simulink model "bh_4bar_model_DYN"  (R2022b)
settings: Solver=ode45  StartTime=0.0  StopTime=10  FixedStep=0.001  MaxStep=0.1  RelTol=1e-9  AbsTol=1e-9  EnableMultiTasking=on
values from neighbouring files (symbols this model uses):
  L1 = 0.4    [bh_4bar_kin_z_analysis_CLS.m]
  L2 = 1.4    [bh_4bar_kin_z_analysis_CLS.m]
  L3 = 1.2    [bh_4bar_kin_z_analysis_CLS.m]
  L4 = 1    [bh_4bar_kin_z_analysis_CLS.m]
  N = length(THE_DEG_ANG_VEC)    [bh_4bar_kin_z_analysis_CLS.m]
  X = my_stuff_T.theta_deg_vec    [bh_4bar_kin_z_analysis_CLS.m]
undefined symbols (not defined in the file or in its folder): alpha_0_rad, alpha_dot_0_rad, alpha_rad, g, H, I_G1, I_G2, I_G3, m1, m2, m3, phi_0_rad, phi_dot_0_rad, phi_rad, theta_0_rad, theta_dot_0_rad, W, Y, Z
libraries: nesl_utility x20, sm_lib x15, simulink_extras x14, bh_4bar_SL_LIB x13
(part 2 of 3)

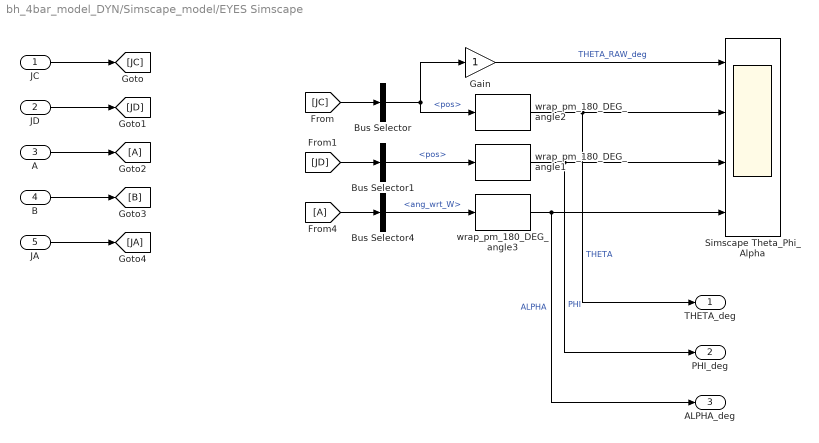
== system bh_4bar_model_DYN/Simscape_model/EYES Simscape ==
  JC : Inport
  JD : Inport  Port=2
  A : Inport  Port=3
  B : Inport  Port=4
  JA : Inport  Port=5
  Bus Selector : BusSelector  OutputSignals=pos
  Bus Selector1 : BusSelector  OutputSignals=pos
  Bus Selector4 : BusSelector  OutputSignals=ang_wrt_W
  From4 : From
  Gain : Gain
  Goto2 : Goto
  Simscape Theta_Phi_Alpha : Scope  NumInputPorts=4
  wrap_pm_180_DEG_angle1 : bh_4bar_SL_LIB/4bar_basics/wrap_pm_180_DEG_angle  SystemSampleTime=-1  VariantActivationTime=update diagram  Latency=0  AutoFrameSizeCalculation=off
  wrap_pm_180_DEG_angle2 : bh_4bar_SL_LIB/4bar_basics/wrap_pm_180_DEG_angle  SystemSampleTime=-1  VariantActivationTime=update diagram  Latency=0  AutoFrameSizeCalculation=off
  wrap_pm_180_DEG_angle3 : bh_4bar_SL_LIB/4bar_basics/wrap_pm_180_DEG_angle  SystemSampleTime=-1  VariantActivationTime=update diagram  Latency=0  AutoFrameSizeCalculation=off
  THETA_deg : Outport  VectorParamsAs1DForOutWhenUnconnected=off
  PHI_deg : Outport  Port=2  VectorParamsAs1DForOutWhenUnconnected=off
  ALPHA_deg : Outport  Port=3  VectorParamsAs1DForOutWhenUnconnected=off
  wires:
  B/1 -> [B]
  A/1 -> Goto2/1
  JD/1 -> [JD]
  JC/1 -> [JC]
  [JD] -> Bus Selector1/1
  [JC] -> Bus Selector/1
  Bus Selector/1 -> wrap_pm_180_DEG_angle2/1, Gain/1  "<pos>"
  From4/1 -> Bus Selector4/1
  wrap_pm_180_DEG_angle2/1 -> THETA_deg/1, Simscape Theta_Phi_Alpha/2  "THETA"
  wrap_pm_180_DEG_angle1/1 -> PHI_deg/1, Simscape Theta_Phi_Alpha/3  "PHI"
  JA/1 -> [JA]
  wrap_pm_180_DEG_angle3/1 -> ALPHA_deg/1, Simscape Theta_Phi_Alpha/4  "ALPHA"
  Gain/1 -> Simscape Theta_Phi_Alpha/1  "THETA_RAW_deg"
  Bus Selector1/1 -> wrap_pm_180_DEG_angle1/1  "<pos>"
  Bus Selector4/1 -> wrap_pm_180_DEG_angle3/1  "<ang_wrt_W>"

== system bh_4bar_model_DYN/Simscape_model/GROUND_C ==
  Mechanism Configuration : sm_lib/Utilities/Mechanism Configuration  UniformGravity=Constant  GravityVector="[0 -g  0]"  GravityUnits=m/s^2  LinearizationDelta=0.001  JointModeTransitionNonlinearIterations=2
  Solver Configuration : nesl_utility/Solver Configuration  PhysicalDomain=network_engine_domain  SubClassName=solver  LeftPortType=input  RightPortType=generic  Tones=[]  Harmonics=[]  SimulateNoise=off  Profile=off  UseLocalSampling=off  EnableSwitchedLinearOptims=on  FrequencyDomain=off  UseCCode=off  RelTol=0.001  AbsTol=1e-06  MinStep=1e-09  ToWorkspace=off  RevertToSquareIcSolve=off  NumHomotopyIterations=100  PhasorMode=off  PhasorModeNumHarmonics=1  ConsistencySolver=NEWTON_FTOL  IndexReductionMethod=DerivativeReplacement  DoDC=off  ResidualTolerance=1e-09  ConsistencyTolSource=GLOBAL  ConsistencyAbsTol=0.001  ConsistencyRelTol=0.001  ConsistencyTolFactor=0.001  UseLocalSolver=off  LocalSolverChoice=NE_BACKWARD_EULER_ADVANCER  ResolveIndetEquations=on  FunctionEvalNumThread=1  LocalSolverSampleTime=0.001  DoFixedCost=off  MaxNonlinIter=3  MaxModeIter=2  ComputeImpulses=off  ImpulseIterations=2  LinearAlgebra=Sparse  LinearAlgebraNumThread=0  EquationFormulation=NE_TIME_EF  DelaysMemoryBudget=1024  AutomaticFiltering=on  FilteringTimeConstant=0.001  PartitionStorageMethod=AS_NEEDED  PartitionMemoryBudget=1024  PartitionMethod=FAST
  World Frame : sm_lib/Frames and Transforms/World Frame
  Conn1 : PMIOPort  Side=Right
  connections:
  Solver Configuration/RConn1 -- Conn1/RConn1 -- Mechanism Configuration/RConn1 -- World Frame/RConn1

== system bh_4bar_model_DYN/Simscape_model/GROUND_D ==
  Rigid Transform : sm_lib/Frames and Transforms/Rigid Transform  TranslationMethod=StandardAxis  TranslationStandardOffset=L4  TranslationLengthUnit=m  TranslationStandardAxis=+X  TranslationCartesianOffset=[0 0 0]  TranslationROffset=0  TranslationROffsetUnits=m  TranslationZOffset=0  TranslationZOffsetUnits=m  TranslationThetaOffset=0  TranslationThetaOffsetUnits=deg  RotationMethod=None  RotationAngleUnits=deg  RotationStandardAxis=+Z  RotationAngle=0.0  RotationArbitraryAxis=[0 0 1]  FollAlignAxisA=+X  BaseAlignAxisA=+Y  FollAlignAxisB=+Y  BaseAlignAxisB=+Z  RotationSequenceAxes=FollowerAxes  RotationSequence=XYX  RotationSequenceAngles=[0 0 0]  RotationSequenceAnglesUnits=deg  RotationMatrix=[1 0 0; 0 1 0; 0 0 1]  Quaternion=[1 0 0 0]
  World Frame1 : sm_lib/Frames and Transforms/World Frame
  Conn1 : PMIOPort  Side=Right
  connections:
  Rigid Transform/LConn1 -- World Frame1/RConn1
  Rigid Transform/RConn1 -- Conn1/RConn1

== system bh_4bar_model_DYN/Simscape_model/Subsystem ==
  THETA_deg : Inport
  PHI_deg : Inport  Port=2
  ALPHA_deg : Inport  Port=3
  Bus Creator : BusCreator  Inputs=3
  ANG_BUS : Outport  VectorParamsAs1DForOutWhenUnconnected=off
  wires:
  ALPHA_deg/1 -> Bus Creator/3  "ALPHA_deg"
  PHI_deg/1 -> Bus Creator/2  "PHI_deg"
  THETA_deg/1 -> Bus Creator/1  "THETA_deg"
  Bus Creator/1 -> ANG_BUS/1

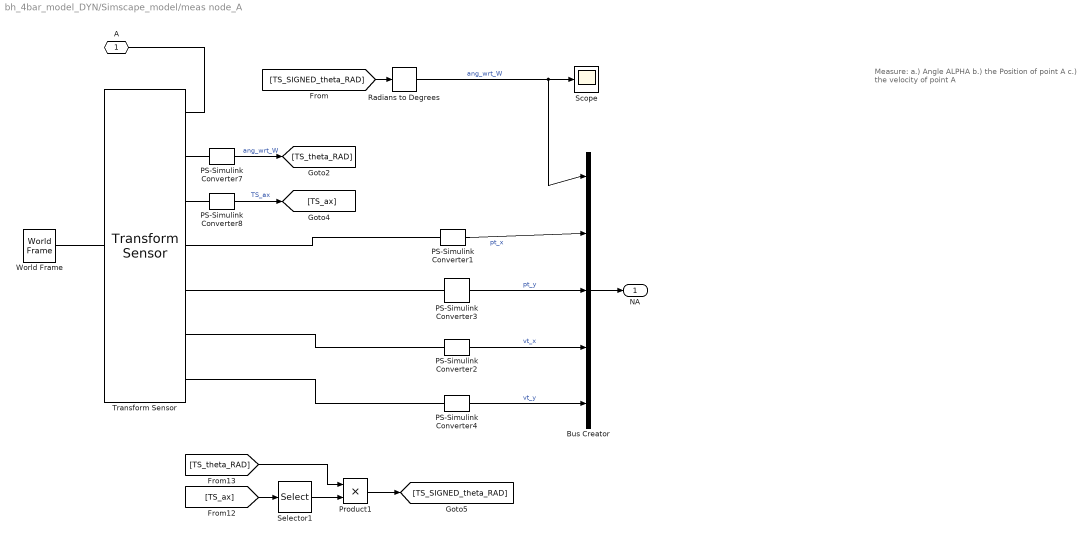
== system bh_4bar_model_DYN/Simscape_model/meas node_A ==
  note: Measure:
      | a.) Angle ALPHA
      | b.) the Position of point A
      | c.) the velocity of point A
  Bus Creator : BusCreator  Inputs=5
  PS-Simulink Converter1 : nesl_utility/PS-Simulink Converter  PhysicalDomain=network_engine_domain  SubClassName=ps_output  LeftPortType=input  RightPortType=output  PseudoPeriodic=off  Frequencies=[]  VectorFormat=1-D array  Unit=m  AffineConversion=off
      settings: AttributesFormatString=UNITS=%<Unit>
  PS-Simulink Converter2 : nesl_utility/PS-Simulink Converter  PhysicalDomain=network_engine_domain  SubClassName=ps_output  LeftPortType=input  RightPortType=output  PseudoPeriodic=off  Frequencies=[]  VectorFormat=1-D array  Unit=m/s  AffineConversion=off
      settings: AttributesFormatString=UNITS=%<Unit>
  PS-Simulink Converter3 : nesl_utility/PS-Simulink Converter  PhysicalDomain=network_engine_domain  SubClassName=ps_output  LeftPortType=input  RightPortType=output  PseudoPeriodic=off  Frequencies=[]  VectorFormat=1-D array  Unit=m  AffineConversion=off
      settings: AttributesFormatString=UNITS=%<Unit>
  PS-Simulink Converter4 : nesl_utility/PS-Simulink Converter  PhysicalDomain=network_engine_domain  SubClassName=ps_output  LeftPortType=input  RightPortType=output  PseudoPeriodic=off  Frequencies=[]  VectorFormat=1-D array  Unit=m/s  AffineConversion=off
      settings: AttributesFormatString=UNITS=%<Unit>
  PS-Simulink Converter7 : nesl_utility/PS-Simulink Converter  PhysicalDomain=network_engine_domain  SubClassName=ps_output  LeftPortType=input  RightPortType=output  PseudoPeriodic=off  Frequencies=[]  VectorFormat=1-D array  Unit=rad  AffineConversion=off
      settings: AttributesFormatString=UNITS=%<Unit>
  PS-Simulink Converter8 : nesl_utility/PS-Simulink Converter  PhysicalDomain=network_engine_domain  SubClassName=ps_output  LeftPortType=input  RightPortType=output  PseudoPeriodic=off  Frequencies=[]  VectorFormat=1-D array  Unit=1  AffineConversion=off
      settings: AttributesFormatString=UNITS=%<Unit>
  Product1 : Product
  Radians to Degrees : simulink_extras/Transformations/Radians to Degrees
  Scope : Scope
  Selector1 : Selector  InputPortWidth=3  IndexOptions=Index vector (dialog)  Indices=3  OutputSizes=1
  Transform Sensor : sm_lib/Frames and Transforms/Transform Sensor  MeasurementFrame=World  SenseAngle=on  SenseAxis=on  SenseQ=off  SenseR=off  SenseRotationSequence=off  RotationSequence=XYX  SenseOmegaX=off  SenseOmegaY=off  SenseOmegaZ=off  SenseQDot=off  SenseRDot=off  SenseAlphaX=off  SenseAlphaY=off  SenseAlphaZ=off  SenseQDDot=off  SenseRDDot=off  SenseX=on  SenseY=on  SenseZ=off  SenseRad=off  SenseAzim=off  SenseDist=off  SenseInc=off  SenseXDot=on  SenseYDot=on  SenseZDot=off  SenseRadDot=off  SenseAzimDot=off  SenseDistDot=off  SenseIncDot=off  SenseXDDot=off  SenseYDDot=off  SenseZDDot=off  SenseRadDDot=off  SenseAzimDDot=off  SenseDistDDot=off  SenseIncDDot=off
  World Frame : sm_lib/Frames and Transforms/World Frame
  A : PMIOPort  Side=Left
  NA : Outport  VectorParamsAs1DForOutWhenUnconnected=off
  wires:
  PS-Simulink Converter2/1 -> Bus Creator/4  "vt_x"
  Bus Creator/1 -> NA/1
  PS-Simulink Converter1/1 -> Bus Creator/2  "pt_x"
  PS-Simulink Converter4/1 -> Bus Creator/5  "vt_y"
  PS-Simulink Converter3/1 -> Bus Creator/3  "pt_y"
  Radians to Degrees/1 -> Bus Creator/1, Scope/1  "ang_wrt_W"
  [TS_theta_RAD] -> Product1/1
  [TS_ax] -> Selector1/1
  Product1/1 -> [TS_SIGNED_theta_RAD]
  Selector1/1 -> Product1/2
  PS-Simulink Converter7/1 -> [TS_theta_RAD]  "ang_wrt_W"
  PS-Simulink Converter8/1 -> [TS_ax]  "TS_ax"
  [TS_SIGNED_theta_RAD] -> Radians to Degrees/1
  connections:
  A/RConn1 -- Transform Sensor/RConn1
  Transform Sensor/LConn1 -- World Frame/RConn1
  Transform Sensor/RConn7 -- PS-Simulink Converter4/LConn1
  PS-Simulink Converter2/LConn1 -- Transform Sensor/RConn6
  PS-Simulink Converter3/LConn1 -- Transform Sensor/RConn5
  PS-Simulink Converter1/LConn1 -- Transform Sensor/RConn4
  PS-Simulink Converter7/LConn1 -- Transform Sensor/RConn2
  PS-Simulink Converter8/LConn1 -- Transform Sensor/RConn3

== system bh_4bar_model_DYN/Simscape_model/meas node_A1 ==
  note: Measure:
      | a.) Angle ALPHA
      | b.) the Position of point A
      | c.) the velocity of point A
  Bus Creator : BusCreator  Inputs=5
  PS-Simulink Converter1 : nesl_utility/PS-Simulink Converter  PhysicalDomain=network_engine_domain  SubClassName=ps_output  LeftPortType=input  RightPortType=output  PseudoPeriodic=off  Frequencies=[]  VectorFormat=1-D array  Unit=m  AffineConversion=off
      settings: AttributesFormatString=UNITS=%<Unit>
  PS-Simulink Converter2 : nesl_utility/PS-Simulink Converter  PhysicalDomain=network_engine_domain  SubClassName=ps_output  LeftPortType=input  RightPortType=output  PseudoPeriodic=off  Frequencies=[]  VectorFormat=1-D array  Unit=m/s  AffineConversion=off
      settings: AttributesFormatString=UNITS=%<Unit>
  PS-Simulink Converter3 : nesl_utility/PS-Simulink Converter  PhysicalDomain=network_engine_domain  SubClassName=ps_output  LeftPortType=input  RightPortType=output  PseudoPeriodic=off  Frequencies=[]  VectorFormat=1-D array  Unit=m  AffineConversion=off
      settings: AttributesFormatString=UNITS=%<Unit>
  PS-Simulink Converter4 : nesl_utility/PS-Simulink Converter  PhysicalDomain=network_engine_domain  SubClassName=ps_output  LeftPortType=input  RightPortType=output  PseudoPeriodic=off  Frequencies=[]  VectorFormat=1-D array  Unit=m/s  AffineConversion=off
      settings: AttributesFormatString=UNITS=%<Unit>
  PS-Simulink Converter7 : nesl_utility/PS-Simulink Converter  PhysicalDomain=network_engine_domain  SubClassName=ps_output  LeftPortType=input  RightPortType=output  PseudoPeriodic=off  Frequencies=[]  VectorFormat=1-D array  Unit=rad  AffineConversion=off
      settings: AttributesFormatString=UNITS=%<Unit>
  PS-Simulink Converter8 : nesl_utility/PS-Simulink Converter  PhysicalDomain=network_engine_domain  SubClassName=ps_output  LeftPortType=input  RightPortType=output  PseudoPeriodic=off  Frequencies=[]  VectorFormat=1-D array  Unit=1  AffineConversion=off
      settings: AttributesFormatString=UNITS=%<Unit>
  Product1 : Product
  Radians to Degrees : simulink_extras/Transformations/Radians to Degrees
  Scope : Scope
  Selector1 : Selector  InputPortWidth=3  IndexOptions=Index vector (dialog)  Indices=3  OutputSizes=1
  Transform Sensor : sm_lib/Frames and Transforms/Transform Sensor  MeasurementFrame=World  SenseAngle=on  SenseAxis=on  SenseQ=off  SenseR=off  SenseRotationSequence=off  RotationSequence=XYX  SenseOmegaX=off  SenseOmegaY=off  SenseOmegaZ=off  SenseQDot=off  SenseRDot=off  SenseAlphaX=off  SenseAlphaY=off  SenseAlphaZ=off  SenseQDDot=off  SenseRDDot=off  SenseX=on  SenseY=on  SenseZ=off  SenseRad=off  SenseAzim=off  SenseDist=off  SenseInc=off  SenseXDot=on  SenseYDot=on  SenseZDot=off  SenseRadDot=off  SenseAzimDot=off  SenseDistDot=off  SenseIncDot=off  SenseXDDot=off  SenseYDDot=off  SenseZDDot=off  SenseRadDDot=off  SenseAzimDDot=off  SenseDistDDot=off  SenseIncDDot=off
  World Frame : sm_lib/Frames and Transforms/World Frame
  B : PMIOPort  Side=Left
  NB : Outport  VectorParamsAs1DForOutWhenUnconnected=off
  wires:
  PS-Simulink Converter2/1 -> Bus Creator/4  "vt_x"
  Bus Creator/1 -> NB/1
  PS-Simulink Converter1/1 -> Bus Creator/2  "pt_x"
  PS-Simulink Converter4/1 -> Bus Creator/5  "vt_y"
  PS-Simulink Converter3/1 -> Bus Creator/3  "pt_y"
  Radians to Degrees/1 -> Bus Creator/1, Scope/1  "ang_wrt_W"
  [TS_theta_RAD] -> Product1/1
  [TS_ax] -> Selector1/1
  Product1/1 -> [TS_SIGNED_theta_RAD]
  Selector1/1 -> Product1/2
  PS-Simulink Converter7/1 -> [TS_theta_RAD]  "ang_wrt_W"
  PS-Simulink Converter8/1 -> [TS_ax]  "TS_ax"
  [TS_SIGNED_theta_RAD] -> Radians to Degrees/1
  connections:
  B/RConn1 -- Transform Sensor/RConn1
  Transform Sensor/LConn1 -- World Frame/RConn1
  Transform Sensor/RConn7 -- PS-Simulink Converter4/LConn1
  PS-Simulink Converter2/LConn1 -- Transform Sensor/RConn6
  PS-Simulink Converter3/LConn1 -- Transform Sensor/RConn5
  PS-Simulink Converter1/LConn1 -- Transform Sensor/RConn4
  PS-Simulink Converter7/LConn1 -- Transform Sensor/RConn2
  PS-Simulink Converter8/LConn1 -- Transform Sensor/RConn3

== system bh_4bar_model_DYN/Simscape_model/meas_JA ==
  Bus Creator : BusCreator  Inputs=2
  PS-Simulink Converter1 : nesl_utility/PS-Simulink Converter  PhysicalDomain=network_engine_domain  SubClassName=ps_output  LeftPortType=input  RightPortType=output  PseudoPeriodic=off  Frequencies=[]  VectorFormat=1-D array  Unit=deg  AffineConversion=off
  PS-Simulink Converter2 : nesl_utility/PS-Simulink Converter  PhysicalDomain=network_engine_domain  SubClassName=ps_output  LeftPortType=input  RightPortType=output  PseudoPeriodic=off  Frequencies=[]  VectorFormat=1-D array  Unit=deg/s  AffineConversion=off
  q : PMIOPort  Side=Left
  w : PMIOPort  Port=2  Side=Left
  PV_BUS : Outport  VectorParamsAs1DForOutWhenUnconnected=off
  wires:
  PS-Simulink Converter2/1 -> Bus Creator/2  "vel"
  PS-Simulink Converter1/1 -> Bus Creator/1  "pos"
  Bus Creator/1 -> PV_BUS/1
  connections:
  q/RConn1 -- PS-Simulink Converter1/LConn1
  PS-Simulink Converter2/LConn1 -- w/RConn1

== system bh_4bar_model_DYN/Simscape_model/meas_JC ==
  Bus Creator : BusCreator  Inputs=2
  PS-Simulink Converter1 : nesl_utility/PS-Simulink Converter  PhysicalDomain=network_engine_domain  SubClassName=ps_output  LeftPortType=input  RightPortType=output  PseudoPeriodic=off  Frequencies=[]  VectorFormat=1-D array  Unit=deg  AffineConversion=off
      settings: AttributesFormatString=UNITS=%<Unit>
  PS-Simulink Converter2 : nesl_utility/PS-Simulink Converter  PhysicalDomain=network_engine_domain  SubClassName=ps_output  LeftPortType=input  RightPortType=output  PseudoPeriodic=off  Frequencies=[]  VectorFormat=1-D array  Unit=deg/s  AffineConversion=off
      settings: AttributesFormatString=UNITS=%<Unit>
  q : PMIOPort  Side=Left
  w : PMIOPort  Port=2  Side=Left
  PV_BUS : Outport  VectorParamsAs1DForOutWhenUnconnected=off
  wires:
  PS-Simulink Converter2/1 -> Bus Creator/2  "vel"
  PS-Simulink Converter1/1 -> Bus Creator/1  "pos"
  Bus Creator/1 -> PV_BUS/1
  connections:
  q/RConn1 -- PS-Simulink Converter1/LConn1
  PS-Simulink Converter2/LConn1 -- w/RConn1

== system bh_4bar_model_DYN/Simscape_model/meas_JD ==
  Bus Creator : BusCreator  Inputs=2
  PS-Simulink Converter1 : nesl_utility/PS-Simulink Converter  PhysicalDomain=network_engine_domain  SubClassName=ps_output  LeftPortType=input  RightPortType=output  PseudoPeriodic=off  Frequencies=[]  VectorFormat=1-D array  Unit=deg  AffineConversion=off
  PS-Simulink Converter2 : nesl_utility/PS-Simulink Converter  PhysicalDomain=network_engine_domain  SubClassName=ps_output  LeftPortType=input  RightPortType=output  PseudoPeriodic=off  Frequencies=[]  VectorFormat=1-D array  Unit=deg/s  AffineConversion=off
  q : PMIOPort  Side=Left
  w : PMIOPort  Port=2  Side=Left
  PV_BUS : Outport  VectorParamsAs1DForOutWhenUnconnected=off
  wires:
  PS-Simulink Converter2/1 -> Bus Creator/2  "vel"
  PS-Simulink Converter1/1 -> Bus Creator/1  "pos"
  Bus Creator/1 -> PV_BUS/1
  connections:
  q/RConn1 -- PS-Simulink Converter1/LConn1
  PS-Simulink Converter2/LConn1 -- w/RConn1

== matlab function bh_4bar_model_DYN/Hand_model/THE_THETA_SYS_DD ==
  data: I_G1 input; theta_DD output; I_G2 input; I_G3 input; L_1 input; L_2 input; L_3 input; alpha input; g input; m_1 input; m_2 input; m_3 input; phi input; tau_1 input; theta input; theta_dot input
function theta_DD = THE_THETA_SYS_DD(I_G1,I_G2,I_G3,L_1,L_2,L_3,alpha,g,m_1,m_2,m_3,phi,tau_1,theta,theta_dot)
%#codegen

%    This function was generated by the Symbolic Math Toolbox version 9.2.
%    27-Oct-2022 15:33:01

et1 = I_G1+I_G3.*((L_1.*cos(alpha).*sin(theta))./(L_3.*(cos(alpha).*sin(phi)-cos(phi).*sin(alpha)))-(L_1.*sin(alpha).*cos(theta))./(L_3.*(cos(alpha).*sin(phi)-cos(phi).*sin(alpha)))).^2+I_G2.*((L_1.*cos(phi).*sin(theta))./(L_2.*(cos(alpha).*sin(phi)-cos(phi).*sin(alpha)))-(L_1.*cos(theta).*sin(phi))./(L_2.*(cos(alpha).*sin(phi)-cos(phi).*sin(alpha)))).^2;
et2 = (m_2.*((L_2.^2.*((L_1.*cos(phi).*sin(theta))./(L_2.*(cos(alpha).*sin(phi)-cos(phi).*sin(alpha)))-(L_1.*cos(theta).*sin(phi))./(L_2.*(cos(alpha).*sin(phi)-cos(phi).*sin(alpha)))).^2)./2.0+L_1.^2.*2.0+L_1.*L_2.*((L_1.*cos(phi).*sin(theta))./(L_2.*(cos(alpha).*sin(phi)-cos(phi).*sin(alpha)))-(L_1.*cos(theta).*sin(phi))./(L_2.*(cos(alpha).*sin(phi)-cos(phi).*sin(alpha)))).*(sin(alpha).*sin(theta)+cos(alpha).*cos(theta)).*2.0))./2.0+(L_1.^2.*m_1)./4.0;
et3 = (L_3.^2.*m_3.*((L_1.*cos(alpha).*sin(theta))./(L_3.*(cos(alpha).*sin(phi)-cos(phi).*sin(alpha)))-(L_1.*sin(alpha).*cos(theta))./(L_3.*(cos(alpha).*sin(phi)-cos(phi).*sin(alpha)))).^2)./4.0;
et4 = cos(alpha).*cos(phi).*((L_1.*cos(phi).*sin(theta))./(L_2.*(cos(alpha).*sin(phi)-cos(phi).*sin(alpha)))-(L_1.*cos(theta).*sin(phi))./(L_2.*(cos(alpha).*sin(phi)-cos(phi).*sin(alpha))))-sin(alpha).*sin(phi).*((L_1.*cos(alpha).*sin(theta))./(L_3.*(cos(alpha).*sin(phi)-cos(phi).*sin(alpha)))-(L_1.*sin(alpha).*cos(theta))./(L_3.*(cos(alpha).*sin(phi)-cos(phi).*sin(alpha))))+sin(alpha).*sin(phi).*((L_1.*cos(phi).*sin(theta))./(L_2.*(cos(alpha).*sin(phi)-cos(phi).*sin(alpha)))-(L_1.*cos(theta).*sin(phi))./(L_2.*(cos(alpha).*sin(phi)-cos(phi).*sin(alpha))));
et5 = -cos(alpha).*cos(phi).*((L_1.*cos(alpha).*sin(theta))./(L_3.*(cos(alpha).*sin(phi)-cos(phi).*sin(alpha)))-(L_1.*sin(alpha).*cos(theta))./(L_3.*(cos(alpha).*sin(phi)-cos(phi).*sin(alpha))));
et6 = cos(alpha).*cos(phi).*((L_1.*cos(phi).*sin(theta))./(L_2.*(cos(alpha).*sin(phi)-cos(phi).*sin(alpha)))-(L_1.*cos(theta).*sin(phi))./(L_2.*(cos(alpha).*sin(phi)-cos(phi).*sin(alpha))))-sin(alpha).*sin(phi).*((L_1.*cos(alpha).*sin(theta))./(L_3.*(cos(alpha).*sin(phi)-cos(phi).*sin(alpha)))-(L_1.*sin(alpha).*cos(theta))./(L_3.*(cos(alpha).*sin(phi)-cos(phi).*sin(alpha))))+sin(alpha).*sin(phi).*((L_1.*cos(phi).*sin(theta))./(L_2.*(cos(alpha).*sin(phi)-cos(phi).*sin(alpha)))-(L_1.*cos(theta).*sin(phi))./(L_2.*(cos(alpha).*sin(phi)-cos(phi).*sin(alpha))));
et7 = -cos(alpha).*cos(phi).*((L_1.*cos(alpha).*sin(theta))./(L_3.*(cos(alpha).*sin(phi)-cos(phi).*sin(alpha)))-(L_1.*sin(alpha).*cos(theta))./(L_3.*(cos(alpha).*sin(phi)-cos(phi).*sin(alpha))));
et8 = (L_1.*cos(phi).*cos(theta))./(L_2.*(cos(alpha).*sin(phi)-cos(phi).*sin(alpha)))+(L_1.*sin(phi).*sin(theta))./(L_2.*(cos(alpha).*sin(phi)-cos(phi).*sin(alpha)))+(L_1.*cos(phi).*sin(theta).*1.0./(cos(alpha).*sin(phi)-cos(phi).*sin(alpha)).^2.*(et4+et5))./L_2-(L_1.*cos(theta).*sin(phi).*1.0./(cos(alpha).*sin(phi)-cos(phi).*sin(alpha)).^2.*(et6+et7))./L_2-(L_1.*cos(phi).*cos(theta).*((L_1.*cos(alpha).*sin(theta))./(L_3.*(cos(alpha).*sin(phi)-cos(phi).*sin(alpha)))-(L_1.*sin(alpha).*cos(theta))./(L_3.*(cos(alpha).*sin(phi)-cos(phi).*sin(alpha)))))./(L_2.*(cos(alpha).*sin(phi)-cos(phi).*sin(alpha)));
et9 = -(L_1.*sin(phi).*sin(theta).*((L_1.*cos(alpha).*sin(theta))./(L_3.*(cos(alpha).*sin(phi)-cos(phi).*sin(alpha)))-(L_1.*sin(alpha).*cos(theta))./(L_3.*(cos(alpha).*sin(phi)-cos(phi).*sin(alpha)))))./(L_2.*(cos(alpha).*sin(phi)-cos(phi).*sin(alpha)));
et10 = cos(alpha).*cos(phi).*((L_1.*cos(phi).*sin(theta))./(L_2.*(cos(alpha).*sin(phi)-cos(phi).*sin(alpha)))-(L_1.*cos(theta).*sin(phi))./(L_2.*(cos(alpha).*sin(phi)-cos(phi).*sin(alpha))))-sin(alpha).*sin(phi).*((L_1.*cos(alpha).*sin(theta))./(L_3.*(cos(alpha).*sin(phi)-cos(phi).*sin(alpha)))-(L_1.*sin(alpha).*cos(theta))./(L_3.*(cos(alpha).*sin(phi)-cos(phi).*sin(alpha))))+sin(alpha).*sin(phi).*((L_1.*cos(phi).*sin(theta))./(L_2.*(cos(alpha).*sin(phi)-cos(phi).*sin(alpha)))-(L_1.*cos(theta).*sin(phi))./(L_2.*(cos(alpha).*sin(phi)-cos(phi).*sin(alpha))));
et11 = -cos(alpha).*cos(phi).*((L_1.*cos(alpha).*sin(theta))./(L_3.*(cos(alpha).*sin(phi)-cos(phi).*sin(alpha)))-(L_1.*sin(alpha).*cos(theta))./(L_3.*(cos(alpha).*sin(phi)-cos(phi).*sin(alpha))));
et12 = cos(alpha).*cos(phi).*((L_1.*cos(phi).*sin(theta))./(L_2.*(cos(alpha).*sin(phi)-cos(phi).*sin(alpha)))-(L_1.*cos(theta).*sin(phi))./(L_2.*(cos(alpha).*sin(phi)-cos(phi).*sin(alpha))))-sin(alpha).*sin(phi).*((L_1.*cos(alpha).*sin(theta))./(L_3.*(cos(alpha).*sin(phi)-cos(phi).*sin(alpha)))-(L_1.*sin(alpha).*cos(theta))./(L_3.*(cos(alpha).*sin(phi)-cos(phi).*sin(alpha))))+sin(alpha).*sin(phi).*((L_1.*cos(phi).*sin(theta))./(L_2.*(cos(alpha).*sin(phi)-cos(phi).*sin(alpha)))-(L_1.*cos(theta).*sin(phi))./(L_2.*(cos(alpha).*sin(phi)-cos(phi).*sin(alpha))));
et13 = -cos(alpha).*cos(phi).*((L_1.*cos(alpha).*sin(theta))./(L_3.*(cos(alpha).*sin(phi)-cos(phi).*sin(alpha)))-(L_1.*sin(alpha).*cos(theta))./(L_3.*(cos(alpha).*sin(phi)-cos(phi).*sin(alpha))));
et14 = (L_1.*cos(phi).*cos(theta))./(L_2.*(cos(alpha).*sin(phi)-cos(phi).*sin(alpha)))+(L_1.*sin(phi).*sin(theta))./(L_2.*(cos(alpha).*sin(phi)-cos(phi).*sin(alpha)))+(L_1.*cos(phi).*sin(theta).*1.0./(cos(alpha).*sin(phi)-cos(phi).*sin(alpha)).^2.*(et10+et11))./L_2-(L_1.*cos(theta).*sin(phi).*1.0./(cos(alpha).*sin(phi)-cos(phi).*sin(alpha)).^2.*(et12+et13))./L_2-(L_1.*cos(phi).*cos(theta).*((L_1.*cos(alpha).*sin(theta))./(L_3.*(cos(alpha).*sin(phi)-cos(phi).*sin(alpha)))-(L_1.*sin(alpha).*cos(theta))./(L_3.*(cos(alpha).*sin(phi)-cos(phi).*sin(alpha)))))./(L_2.*(cos(alpha).*sin(phi)-cos(phi).*sin(alpha)));
et15 = -(L_1.*sin(phi).*sin(theta).*((L_1.*cos(alpha).*sin(theta))./(L_3.*(cos(alpha).*sin(phi)-cos(phi).*sin(alpha)))-(L_1.*sin(alpha).*cos(theta))./(L_3.*(cos(alpha).*sin(phi)-cos(phi).*sin(alpha)))))./(L_2.*(cos(alpha).*sin(phi)-cos(phi).*sin(alpha)));
et16 = (L_2.^2.*theta_dot.^2.*((L_1.*cos(phi).*sin(theta))./(L_2.*(cos(alpha).*sin(phi)-cos(phi).*sin(alpha)))-(L_1.*cos(theta).*sin(phi))./(L_2.*(cos(alpha).*sin(phi)-cos(phi).*sin(alpha)))).*(et8+et9))./2.0+L_1.*L_2.*theta_dot.^2.*(sin(alpha).*sin(theta)+cos(alpha).*cos(theta)).*(et14+et15);
et17 = -L_1.*L_2.*theta_dot.^2.*((L_1.*cos(phi).*sin(theta))./(L_2.*(cos(alpha).*sin(phi)-cos(phi).*sin(alpha)))-(L_1.*cos(theta).*sin(phi))./(L_2.*(cos(alpha).*sin(phi)-cos(phi).*sin(alpha)))).*(cos(alpha).*sin(theta)-sin(alpha).*cos(theta)-cos(alpha).*sin(theta).*((L_1.*cos(phi).*sin(theta))./(L_2.*(cos(alpha).*sin(phi)-cos(phi).*sin(alpha)))-(L_1.*cos(theta).*sin(phi))./(L_2.*(cos(alpha).*sin(phi)-cos(phi).*sin(alpha))))+sin(alpha).*cos(theta).*((L_1.*cos(phi).*sin(theta))./(L_2.*(cos(alpha).*sin(phi)-cos(phi).*sin(alpha)))-(L_1.*cos(theta).*sin(phi))./(L_2.*(cos(alpha).*sin(phi)-cos(phi).*sin(alpha)))));
et18 = theta_dot.*cos(alpha).*cos(phi).*((L_1.*cos(alpha).*sin(theta))./(L_3.*(cos(alpha).*sin(phi)-cos(phi).*sin(alpha)))-(L_1.*sin(alpha).*cos(theta))./(L_3.*(cos(alpha).*sin(phi)-cos(phi).*sin(alpha))))-theta_dot.*cos(alpha).*cos(phi).*((L_1.*cos(phi).*sin(theta))./(L_2.*(cos(alpha).*sin(phi)-cos(phi).*sin(alpha)))-(L_1.*cos(theta).*sin(phi))./(L_2.*(cos(alpha).*sin(phi)-cos(phi).*sin(alpha))))+theta_dot.*sin(alpha).*sin(phi).*((L_1.*cos(alpha).*sin(theta))./(L_3.*(cos(alpha).*sin(phi)-cos(phi).*sin(alpha)))-(L_1.*sin(alpha).*cos(theta))./(L_3.*(cos(alpha).*sin(phi)-cos(phi).*sin(alpha))));
et19 = -theta_dot.*sin(alpha).*sin(phi).*((L_1.*cos(phi).*sin(theta))./(L_2.*(cos(alpha).*sin(phi)-cos(phi).*sin(alpha)))-(L_1.*cos(theta).*sin(phi))./(L_2.*(cos(alpha).*sin(phi)-cos(phi).*sin(alpha))));
et20 = theta_dot.*cos(alpha).*cos(phi).*((L_1.*cos(alpha).*sin(theta))./(L_3.*(cos(alpha).*sin(phi)-cos(phi).*sin(alpha)))-(L_1.*sin(alpha).*cos(theta))./(L_3.*(cos(alpha).*sin(phi)-cos(phi).*sin(alpha))))-theta_dot.*cos(alpha).*cos(phi).*((L_1.*cos(phi).*sin(theta))./(L_2.*(cos(alpha).*sin(phi)-cos(phi).*sin(alpha)))-(L_1.*cos(theta).*sin(phi))./(L_2.*(cos(alpha).*sin(phi)-cos(phi).*sin(alpha))))+theta_dot.*sin(alpha).*sin(phi).*((L_1.*cos(alpha).*sin(theta))./(L_3.*(cos(alpha).*sin(phi)-cos(phi).*sin(alpha)))-(L_1.*sin(alpha).*cos(theta))./(L_3.*(cos(alpha).*sin(phi)-cos(phi).*sin(alpha))));
et21 = -theta_dot.*sin(alpha).*sin(phi).*((L_1.*cos(phi).*sin(theta))./(L_2.*(cos(alpha).*sin(phi)-cos(phi).*sin(alpha)))-(L_1.*cos(theta).*sin(phi))./(L_2.*(cos(alpha).*sin(phi)-cos(phi).*sin(alpha))));
et22 = (L_1.*theta_dot.*cos(phi).*cos(theta))./(L_2.*(cos(alpha).*sin(phi)-cos(phi).*sin(alpha)))+(L_1.*theta_dot.*sin(phi).*sin(theta))./(L_2.*(cos(alpha).*sin(phi)-cos(phi).*sin(alpha)))-(L_1.*cos(phi).*sin(theta).*1.0./(cos(alpha).*sin(phi)-cos(phi).*sin(alpha)).^2.*(et18+et19))./L_2+(L_1.*cos(theta).*sin(phi).*1.0./(cos(alpha).*sin(phi)-cos(phi).*sin(alpha)).^2.*(et20+et21))./L_2-(L_1.*theta_dot.*cos(phi).*cos(theta).*((L_1.*cos(alpha).*sin(theta))./(L_3.*(cos(alpha).*sin(phi)-cos(phi).*sin(alpha)))-(L_1.*sin(alpha).*cos(theta))./(L_3.*(cos(alpha).*sin(phi)-cos(phi).*sin(alpha)))))./(L_2.*(cos(alpha).*sin(phi)-cos(phi).*sin(alpha)));
et23 = -(L_1.*theta_dot.*sin(phi).*sin(theta).*((L_1.*cos(alpha).*sin(theta))./(L_3.*(cos(alpha).*sin(phi)-cos(phi).*sin(alpha)))-(L_1.*sin(alpha).*cos(theta))./(L_3.*(cos(alpha).*sin(phi)-cos(phi).*sin(alpha)))))./(L_2.*(cos(alpha).*sin(phi)-cos(phi).*sin(alpha)));
et24 = theta_dot.*cos(alpha).*cos(phi).*((L_1.*cos(alpha).*sin(theta))./(L_3.*(cos(alpha).*sin(phi)-cos(phi).*sin(alpha)))-(L_1.*sin(alpha).*cos(theta))./(L_3.*(cos(alpha).*sin(phi)-cos(phi).*sin(alpha))))-theta_dot.*cos(alpha).*cos(phi).*((L_1.*cos(phi).*sin(theta))./(L_2.*(cos(alpha).*sin(phi)-cos(phi).*sin(alpha)))-(L_1.*cos(theta).*sin(phi))./(L_2.*(cos(alpha).*sin(phi)-cos(phi).*sin(alpha))))+theta_dot.*sin(alpha).*sin(phi).*((L_1.*cos(alpha).*sin(theta))./(L_3.*(cos(alpha).*sin(phi)-cos(phi).*sin(alpha)))-(L_1.*sin(alpha).*cos(theta))./(L_3.*(cos(alpha).*sin(phi)-cos(phi).*sin(alpha))));
et25 = -theta_dot.*sin(alpha).*sin(phi).*((L_1.*cos(phi).*sin(theta))./(L_2.*(cos(alpha).*sin(phi)-cos(phi).*sin(alpha)))-(L_1.*cos(theta).*sin(phi))./(L_2.*(cos(alpha).*sin(phi)-cos(phi).*sin(alpha))));
et26 = theta_dot.*cos(alpha).*cos(phi).*((L_1.*cos(alpha).*sin(theta))./(L_3.*(cos(alpha).*sin(phi)-cos(phi).*sin(alpha)))-(L_1.*sin(alpha).*cos(theta))./(L_3.*(cos(alpha).*sin(phi)-cos(phi).*sin(alpha))))-theta_dot.*cos(alpha).*cos(phi).*((L_1.*cos(phi).*sin(theta))./(L_2.*(cos(alpha).*sin(phi)-cos(phi).*sin(alpha)))-(L_1.*cos(theta).*sin(phi))./(L_2.*(cos(alpha).*sin(phi)-cos(phi).*sin(alpha))))+theta_dot.*sin(alpha).*sin(phi).*((L_1.*cos(alpha).*sin(theta))./(L_3.*(cos(alpha).*sin(phi)-cos(phi).*sin(alpha)))-(L_1.*sin(alpha).*cos(theta))./(L_3.*(cos(alpha).*sin(phi)-cos(phi).*sin(alpha))));
et27 = -theta_dot.*sin(alpha).*sin(phi).*((L_1.*cos(phi).*sin(theta))./(L_2.*(cos(alpha).*sin(phi)-cos(phi).*sin(alpha)))-(L_1.*cos(theta).*sin(phi))./(L_2.*(cos(alpha).*sin(phi)-cos(phi).*sin(alpha))));
et28 = (L_1.*theta_dot.*cos(phi).*cos(theta))./(L_2.*(cos(alpha).*sin(phi)-cos(phi).*sin(alpha)))+(L_1.*theta_dot.*sin(phi).*sin(theta))./(L_2.*(cos(alpha).*sin(phi)-cos(phi).*sin(alpha)))-(L_1.*cos(phi).*sin(theta).*1.0./(cos(alpha).*sin(phi)-cos(phi).*sin(alpha)).^2.*(et24+et25))./L_2+(L_1.*cos(theta).*sin(phi).*1.0./(cos(alpha).*sin(phi)-cos(phi).*sin(alpha)).^2.*(et26+et27))./L_2-(L_1.*theta_dot.*cos(phi).*cos(theta).*((L_1.*cos(alpha).*sin(theta))./(L_3.*(cos(alpha).*sin(phi)-cos(phi).*sin(alpha)))-(L_1.*sin(alpha).*cos(theta))./(L_3.*(cos(alpha).*sin(phi)-cos(phi).*sin(alpha)))))./(L_2.*(cos(alpha).*sin(phi)-cos(phi).*sin(alpha)));
et29 = -(L_1.*theta_dot.*sin(phi).*sin(theta).*((L_1.*cos(alpha).*sin(theta))./(L_3.*(cos(alpha).*sin(phi)-cos(phi).*sin(alpha)))-(L_1.*sin(alpha).*cos(theta))./(L_3.*(cos(alpha).*sin(phi)-cos(phi).*sin(alpha)))))./(L_2.*(cos(alpha).*sin(phi)-cos(phi).*sin(alpha)));
et30 = L_2.^2.*theta_dot.*((L_1.*cos(phi).*sin(theta))./(L_2.*(cos(alpha).*sin(phi)-cos(phi).*sin(alpha)))-(L_1.*cos(theta).*sin(phi))./(L_2.*(cos(alpha).*sin(phi)-cos(phi).*sin(alpha)))).*(et22+et23);
et31 = L_1.*L_2.*theta_dot.*((L_1.*cos(phi).*sin(theta))./(L_2.*(cos(alpha).*sin(phi)-cos(phi).*sin(alpha)))-(L_1.*cos(theta).*sin(phi))./(L_2.*(cos(alpha).*sin(phi)-cos(phi).*sin(alpha)))).*(theta_dot.*cos(alpha).*sin(theta)-theta_dot.*sin(alpha).*cos(theta)-theta_dot.*cos(alpha).*sin(theta).*((L_1.*cos(phi).*sin(theta))./(L_2.*(cos(alpha).*sin(phi)-cos(phi).*sin(alpha)))-(L_1.*cos(theta).*sin(phi))./(L_2.*(cos(alpha).*sin(phi)-cos(phi).*sin(alpha))))+theta_dot.*sin(alpha).*cos(theta).*((L_1.*cos(phi).*sin(theta))./(L_2.*(cos(alpha).*sin(phi)-cos(phi).*sin(alpha)))-(L_1.*cos(theta).*sin(phi))./(L_2.*(cos(alpha).*sin(phi)-cos(phi).*sin(alpha))))).*-2.0;
et32 = L_1.*L_2.*theta_dot.*(sin(alpha).*sin(theta)+cos(alpha).*cos(theta)).*(et28+et29).*2.0;
et33 = cos(alpha).*cos(phi).*((L_1.*cos(phi).*sin(theta))./(L_2.*(cos(alpha).*sin(phi)-cos(phi).*sin(alpha)))-(L_1.*cos(theta).*sin(phi))./(L_2.*(cos(alpha).*sin(phi)-cos(phi).*sin(alpha))))-sin(alpha).*sin(phi).*((L_1.*cos(alpha).*sin(theta))./(L_3.*(cos(alpha).*sin(phi)-cos(phi).*sin(alpha)))-(L_1.*sin(alpha).*cos(theta))./(L_3.*(cos(alpha).*sin(phi)-cos(phi).*sin(alpha))))+sin(alpha).*sin(phi).*((L_1.*cos(phi).*sin(theta))./(L_2.*(cos(alpha).*sin(phi)-cos(phi).*sin(alpha)))-(L_1.*cos(theta).*sin(phi))./(L_2.*(cos(alpha).*sin(phi)-cos(phi).*sin(alpha))));
et34 = -cos(alpha).*cos(phi).*((L_1.*cos(alpha).*sin(theta))./(L_3.*(cos(alpha).*sin(phi)-cos(phi).*sin(alpha)))-(L_1.*sin(alpha).*cos(theta))./(L_3.*(cos(alpha).*sin(phi)-cos(phi).*sin(alpha))));
et35 = cos(alpha).*cos(phi).*((L_1.*cos(phi).*sin(theta))./(L_2.*(cos(alpha).*sin(phi)-cos(phi).*sin(alpha)))-(L_1.*cos(theta).*sin(phi))./(L_2.*(cos(alpha).*sin(phi)-cos(phi).*sin(alpha))))-sin(alpha).*sin(phi).*((L_1.*cos(alpha).*sin(theta))./(L_3.*(cos(alpha).*sin(phi)-cos(phi).*sin(alpha)))-(L_1.*sin(alpha).*cos(theta))./(L_3.*(cos(alpha).*sin(phi)-cos(phi).*sin(alpha))))+sin(alpha).*sin(phi).*((L_1.*cos(phi).*sin(theta))./(L_2.*(cos(alpha).*sin(phi)-cos(phi).*sin(alpha)))-(L_1.*cos(theta).*sin(phi))./(L_2.*(cos(alpha).*sin(phi)-cos(phi).*sin(alpha))));
et36 = -cos(alpha).*cos(phi).*((L_1.*cos(alpha).*sin(theta))./(L_3.*(cos(alpha).*sin(phi)-cos(phi).*sin(alpha)))-(L_1.*sin(alpha).*cos(theta))./(L_3.*(cos(alpha).*sin(phi)-cos(phi).*sin(alpha))));
et37 = (L_1.*cos(phi).*cos(theta))./(L_2.*(cos(alpha).*sin(phi)-cos(phi).*sin(alpha)))+(L_1.*sin(phi).*sin(theta))./(L_2.*(cos(alpha).*sin(phi)-cos(phi).*sin(alpha)))+(L_1.*cos(phi).*sin(theta).*1.0./(cos(alpha).*sin(phi)-cos(phi).*sin(alpha)).^2.*(et33+et34))./L_2-(L_1.*cos(theta).*sin(phi).*1.0./(cos(alpha).*sin(phi)-cos(phi).*sin(alpha)).^2.*(et35+et36))./L_2-(L_1.*cos(phi).*cos(theta).*((L_1.*cos(alpha).*sin(theta))./(L_3.*(cos(alpha).*sin(phi)-cos(phi).*sin(alpha)))-(L_1.*sin(alpha).*cos(theta))./(L_3.*(cos(alpha).*sin(phi)-cos(phi).*sin(alpha)))))./(L_2.*(cos(alpha).*sin(phi)-cos(phi).*sin(alpha)));
et38 = -(L_1.*sin(phi).*sin(theta).*((L_1.*cos(alpha).*sin(theta))./(L_3.*(cos(alpha).*sin(phi)-cos(phi).*sin(alpha)))-(L_1.*sin(alpha).*cos(theta))./(L_3.*(cos(alpha).*sin(phi)-cos(phi).*sin(alpha)))))./(L_2.*(cos(alpha).*sin(phi)-cos(phi).*sin(alpha)));
et39 = theta_dot.*cos(alpha).*cos(phi).*((L_1.*cos(alpha).*sin(theta))./(L_3.*(cos(alpha).*sin(phi)-cos(phi).*sin(alpha)))-(L_1.*sin(alpha).*cos(theta))./(L_3.*(cos(alpha).*sin(phi)-cos(phi).*sin(alpha))))-theta_dot.*cos(alpha).*cos(phi).*((L_1.*cos(phi).*sin(theta))./(L_2.*(cos(alpha).*sin(phi)-cos(phi).*sin(alpha)))-(L_1.*cos(theta).*sin(phi))./(L_2.*(cos(alpha).*sin(phi)-cos(phi).*sin(alpha))))+theta_dot.*sin(alpha).*sin(phi).*((L_1.*cos(alpha).*sin(theta))./(L_3.*(cos(alpha).*sin(phi)-cos(phi).*sin(alpha)))-(L_1.*sin(alpha).*cos(theta))./(L_3.*(cos(alpha).*sin(phi)-cos(phi).*sin(alpha))));
et40 = -theta_dot.*sin(alpha).*sin(phi).*((L_1.*cos(phi).*sin(theta))./(L_2.*(cos(alpha).*sin(phi)-cos(phi).*sin(alpha)))-(L_1.*cos(theta).*sin(phi))./(L_2.*(cos(alpha).*sin(phi)-cos(phi).*sin(alpha))));
et41 = theta_dot.*cos(alpha).*cos(phi).*((L_1.*cos(alpha).*sin(theta))./(L_3.*(cos(alpha).*sin(phi)-cos(phi).*sin(alpha)))-(L_1.*sin(alpha).*cos(theta))./(L_3.*(cos(alpha).*sin(phi)-cos(phi).*sin(alpha))))-theta_dot.*cos(alpha).*cos(phi).*((L_1.*cos(phi).*sin(theta))./(L_2.*(cos(alpha).*sin(phi)-cos(phi).*sin(alpha)))-(L_1.*cos(theta).*sin(phi))./(L_2.*(cos(alpha).*sin(phi)-cos(phi).*sin(alpha))))+theta_dot.*sin(alpha).*sin(phi).*((L_1.*cos(alpha).*sin(theta))./(L_3.*(cos(alpha).*sin(phi)-cos(phi).*sin(alpha)))-(L_1.*sin(alpha).*cos(theta))./(L_3.*(cos(alpha).*sin(phi)-cos(phi).*sin(alpha))));
et42 = -theta_dot.*sin(alpha).*sin(phi).*((L_1.*cos(phi).*sin(theta))./(L_2.*(cos(alpha).*sin(phi)-cos(phi).*sin(alpha)))-(L_1.*cos(theta).*sin(phi))./(L_2.*(cos(alpha).*sin(phi)-cos(phi).*sin(alpha))));
et43 = (L_1.*theta_dot.*cos(phi).*cos(theta))./(L_2.*(cos(alpha).*sin(phi)-cos(phi).*sin(alpha)))+(L_1.*theta_dot.*sin(phi).*sin(theta))./(L_2.*(cos(alpha).*sin(phi)-cos(phi).*sin(alpha)))-(L_1.*cos(phi).*sin(theta).*1.0./(cos(alpha).*sin(phi)-cos(phi).*sin(alpha)).^2.*(et39+et40))./L_2+(L_1.*cos(theta).*sin(phi).*1.0./(cos(alpha).*sin(phi)-cos(phi).*sin(alpha)).^2.*(et41+et42))./L_2-(L_1.*theta_dot.*cos(phi).*cos(theta).*((L_1.*cos(alpha).*sin(theta))./(L_3.*(cos(alpha).*sin(phi)-cos(phi).*sin(alpha)))-(L_1.*sin(alpha).*cos(theta))./(L_3.*(cos(alpha).*sin(phi)-cos(phi).*sin(alpha)))))./(L_2.*(cos(alpha).*sin(phi)-cos(phi).*sin(alpha)));
et44 = -(L_1.*theta_dot.*sin(phi).*sin(theta).*((L_1.*cos(alpha).*sin(theta))./(L_3.*(cos(alpha).*sin(phi)-cos(phi).*sin(alpha)))-(L_1.*sin(alpha).*cos(theta))./(L_3.*(cos(alpha).*sin(phi)-cos(phi).*sin(alpha)))))./(L_2.*(cos(alpha).*sin(phi)-cos(phi).*sin(alpha)));
et45 = cos(alpha).*cos(phi).*((L_1.*cos(phi).*sin(theta))./(L_2.*(cos(alpha).*sin(phi)-cos(phi).*sin(alpha)))-(L_1.*cos(theta).*sin(phi))./(L_2.*(cos(alpha).*sin(phi)-cos(phi).*sin(alpha))))-sin(alpha).*sin(phi).*((L_1.*cos(alpha).*sin(theta))./(L_3.*(cos(alpha).*sin(phi)-cos(phi).*sin(alpha)))-(L_1.*sin(alpha).*cos(theta))./(L_3.*(cos(alpha).*sin(phi)-cos(phi).*sin(alpha))))+sin(alpha).*sin(phi).*((L_1.*cos(phi).*sin(theta))./(L_2.*(cos(alpha).*sin(phi)-cos(phi).*sin(alpha)))-(L_1.*cos(theta).*sin(phi))./(L_2.*(cos(alpha).*sin(phi)-cos(phi).*sin(alpha))));
et46 = -cos(alpha).*cos(phi).*((L_1.*cos(alpha).*sin(theta))./(L_3.*(cos(alpha).*sin(phi)-cos(phi).*sin(alpha)))-(L_1.*sin(alpha).*cos(theta))./(L_3.*(cos(alpha).*sin(phi)-cos(phi).*sin(alpha))));
et47 = cos(alpha).*cos(phi).*((L_1.*cos(phi).*sin(theta))./(L_2.*(cos(alpha).*sin(phi)-cos(phi).*sin(alpha)))-(L_1.*cos(theta).*sin(phi))./(L_2.*(cos(alpha).*sin(phi)-cos(phi).*sin(alpha))))-sin(alpha).*sin(phi).*((L_1.*cos(alpha).*sin(theta))./(L_3.*(cos(alpha).*sin(phi)-cos(phi).*sin(alpha)))-(L_1.*sin(alpha).*cos(theta))./(L_3.*(cos(alpha).*sin(phi)-cos(phi).*sin(alpha))))+sin(alpha).*sin(phi).*((L_1.*cos(phi).*sin(theta))./(L_2.*(cos(alpha).*sin(phi)-cos(phi).*sin(alpha)))-(L_1.*cos(theta).*sin(phi))./(L_2.*(cos(alpha).*sin(phi)-cos(phi).*sin(alpha))));
et48 = -cos(alpha).*cos(phi).*((L_1.*cos(alpha).*sin(theta))./(L_3.*(cos(alpha).*sin(phi)-cos(phi).*sin(alpha)))-(L_1.*sin(alpha).*cos(theta))./(L_3.*(cos(alpha).*sin(phi)-cos(phi).*sin(alpha))));
et49 = (L_1.*cos(alpha).*cos(theta))./(L_3.*(cos(alpha).*sin(phi)-cos(phi).*sin(alpha)))+(L_1.*sin(alpha).*sin(theta))./(L_3.*(cos(alpha).*sin(phi)-cos(phi).*sin(alpha)))-(L_1.*sin(alpha).*sin(theta).*((L_1.*cos(phi).*sin(theta))./(L_2.*(cos(alpha).*sin(phi)-cos(phi).*sin(alpha)))-(L_1.*cos(theta).*sin(phi))./(L_2.*(cos(alpha).*sin(phi)-cos(phi).*sin(alpha)))))./(L_3.*(cos(alpha).*sin(phi)-cos(phi).*sin(alpha)))+(L_1.*cos(alpha).*sin(theta).*1.0./(cos(alpha).*sin(phi)-cos(phi).*sin(alpha)).^2.*(et45+et46))./L_3-(L_1.*sin(alpha).*cos(theta).*1.0./(cos(alpha).*sin(phi)-cos(phi).*sin(alpha)).^2.*(et47+et48))./L_3;
et50 = -(L_1.*cos(alpha).*cos(theta).*((L_1.*cos(phi).*sin(theta))./(L_2.*(cos(alpha).*sin(phi)-cos(phi).*sin(alpha)))-(L_1.*cos(theta).*sin(phi))./(L_2.*(cos(alpha).*sin(phi)-cos(phi).*sin(alpha)))))./(L_3.*(cos(alpha).*sin(phi)-cos(phi).*sin(alpha)));
et51 = theta_dot.*cos(alpha).*cos(phi).*((L_1.*cos(alpha).*sin(theta))./(L_3.*(cos(alpha).*sin(phi)-cos(phi).*sin(alpha)))-(L_1.*sin(alpha).*cos(theta))./(L_3.*(cos(alpha).*sin(phi)-cos(phi).*sin(alpha))))-theta_dot.*cos(alpha).*cos(phi).*((L_1.*cos(phi).*sin(theta))./(L_2.*(cos(alpha).*sin(phi)-cos(phi).*sin(alpha)))-(L_1.*cos(theta).*sin(phi))./(L_2.*(cos(alpha).*sin(phi)-cos(phi).*sin(alpha))))+theta_dot.*sin(alpha).*sin(phi).*((L_1.*cos(alpha).*sin(theta))./(L_3.*(cos(alpha).*sin(phi)-cos(phi).*sin(alpha)))-(L_1.*sin(alpha).*cos(theta))./(L_3.*(cos(alpha).*sin(phi)-cos(phi).*sin(alpha))));
et52 = -theta_dot.*sin(alpha).*sin(phi).*((L_1.*cos(phi).*sin(theta))./(L_2.*(cos(alpha).*sin(phi)-cos(phi).*sin(alpha)))-(L_1.*cos(theta).*sin(phi))./(L_2.*(cos(alpha).*sin(phi)-cos(phi).*sin(alpha))));
et53 = theta_dot.*cos(alpha).*cos(phi).*((L_1.*cos(alpha).*sin(theta))./(L_3.*(cos(alpha).*sin(phi)-cos(phi).*sin(alpha)))-(L_1.*sin(alpha).*cos(theta))./(L_3.*(cos(alpha).*sin(phi)-cos(phi).*sin(alpha))))-theta_dot.*cos(alpha).*cos(phi).*((L_1.*cos(phi).*sin(theta))./(L_2.*(cos(alpha).*sin(phi)-cos(phi).*sin(alpha)))-(L_1.*cos(theta).*sin(phi))./(L_2.*(cos(alpha).*sin(phi)-cos(phi).*sin(alpha))))+theta_dot.*sin(alpha).*sin(phi).*((L_1.*cos(alpha).*sin(theta))./(L_3.*(cos(alpha).*sin(phi)-cos(phi).*sin(alpha)))-(L_1.*sin(alpha).*cos(theta))./(L_3.*(cos(alpha).*sin(phi)-cos(phi).*sin(alpha))));
et54 = -theta_dot.*sin(alpha).*sin(phi).*((L_1.*cos(phi).*sin(theta))./(L_2.*(cos(alpha).*sin(phi)-cos(phi).*sin(alpha)))-(L_1.*cos(theta).*sin(phi))./(L_2.*(cos(alpha).*sin(phi)-cos(phi).*sin(alpha))));
et55 = (L_1.*theta_dot.*cos(alpha).*cos(theta))./(L_3.*(cos(alpha).*sin(phi)-cos(phi).*sin(alpha)))+(L_1.*theta_dot.*sin(alpha).*sin(theta))./(L_3.*(cos(alpha).*sin(phi)-cos(phi).*sin(alpha)))-(L_1.*cos(alpha).*sin(theta).*1.0./(cos(alpha).*sin(phi)-cos(phi).*sin(alpha)).^2.*(et51+et52))./L_3+(L_1.*sin(alpha).*cos(theta).*1.0./(cos(alpha).*sin(phi)-cos(phi).*sin(alpha)).^2.*(et53+et54))./L_3-(L_1.*theta_dot.*cos(alpha).*cos(theta).*((L_1.*cos(phi).*sin(theta))./(L_2.*(cos(alpha).*sin(phi)-cos(phi).*sin(alpha)))-(L_1.*cos(theta).*sin(phi))./(L_2.*(cos(alpha).*sin(phi)-cos(phi).*sin(alpha)))))./(L_3.*(cos(alpha).*sin(phi)-cos(phi).*sin(alpha)));
et56 = -(L_1.*theta_dot.*sin(alpha).*sin(theta).*((L_1.*cos(phi).*sin(theta))./(L_2.*(cos(alpha).*sin(phi)-cos(phi).*sin(alpha)))-(L_1.*cos(theta).*sin(phi))./(L_2.*(cos(alpha).*sin(phi)-cos(phi).*sin(alpha)))))./(L_3.*(cos(alpha).*sin(phi)-cos(phi).*sin(alpha)));
et57 = cos(alpha).*cos(phi).*((L_1.*cos(phi).*sin(theta))./(L_2.*(cos(alpha).*sin(phi)-cos(phi).*sin(alpha)))-(L_1.*cos(theta).*sin(phi))./(L_2.*(cos(alpha).*sin(phi)-cos(phi).*sin(alpha))))-sin(alpha).*sin(phi).*((L_1.*cos(alpha).*sin(theta))./(L_3.*(cos(alpha).*sin(phi)-cos(phi).*sin(alpha)))-(L_1.*sin(alpha).*cos(theta))./(L_3.*(cos(alpha).*sin(phi)-cos(phi).*sin(alpha))))+sin(alpha).*sin(phi).*((L_1.*cos(phi).*sin(theta))./(L_2.*(cos(alpha).*sin(phi)-cos(phi).*sin(alpha)))-(L_1.*cos(theta).*sin(phi))./(L_2.*(cos(alpha).*sin(phi)-cos(phi).*sin(alpha))));
et58 = -cos(alpha).*cos(phi).*((L_1.*cos(alpha).*sin(theta))./(L_3.*(cos(alpha).*sin(phi)-cos(phi).*sin(alpha)))-(L_1.*sin(alpha).*cos(theta))./(L_3.*(cos(alpha).*sin(phi)-cos(phi).*sin(alpha))));
et59 = cos(alpha).*cos(phi).*((L_1.*cos(phi).*sin(theta))./(L_2.*(cos(alpha).*sin(phi)-cos(phi).*sin(alpha)))-(L_1.*cos(theta).*sin(phi))./(L_2.*(cos(alpha).*sin(phi)-cos(phi).*sin(alpha))))-sin(alpha).*sin(phi).*((L_1.*cos(alpha).*sin(theta))./(L_3.*(cos(alpha).*sin(phi)-cos(phi).*sin(alpha)))-(L_1.*sin(alpha).*cos(theta))./(L_3.*(cos(alpha).*sin(phi)-cos(phi).*sin(alpha))))+sin(alpha).*sin(phi).*((L_1.*cos(phi).*sin(theta))./(L_2.*(cos(alpha).*sin(phi)-cos(phi).*sin(alpha)))-(L_1.*cos(theta).*sin(phi))./(L_2.*(cos(alpha).*sin(phi)-cos(phi).*sin(alpha))));
et60 = -cos(alpha).*cos(phi).*((L_1.*cos(alpha).*sin(theta))./(L_3.*(cos(alpha).*sin(phi)-cos(phi).*sin(alpha)))-(L_1.*sin(alpha).*cos(theta))./(L_3.*(cos(alpha).*sin(phi)-cos(phi).*sin(alpha))));
et61 = (L_1.*cos(alpha).*cos(theta))./(L_3.*(cos(alpha).*sin(phi)-cos(phi).*sin(alpha)))+(L_1.*sin(alpha).*sin(theta))./(L_3.*(cos(alpha).*sin(phi)-cos(phi).*sin(alpha)))-(L_1.*sin(alpha).*sin(theta).*((L_1.*cos(phi).*sin(theta))./(L_2.*(cos(alpha).*sin(phi)-cos(phi).*sin(alpha)))-(L_1.*cos(theta).*sin(phi))./(L_2.*(cos(alpha).*sin(phi)-cos(phi).*sin(alpha)))))./(L_3.*(cos(alpha).*sin(phi)-cos(phi).*sin(alpha)))+(L_1.*cos(alpha).*sin(theta).*1.0./(cos(alpha).*sin(phi)-cos(phi).*sin(alpha)).^2.*(et57+et58))./L_3-(L_1.*sin(alpha).*cos(theta).*1.0./(cos(alpha).*sin(phi)-cos(phi).*sin(alpha)).^2.*(et59+et60))./L_3;
et62 = -(L_1.*cos(alpha).*cos(theta).*((L_1.*cos(phi).*sin(theta))./(L_2.*(cos(alpha).*sin(phi)-cos(phi).*sin(alpha)))-(L_1.*cos(theta).*sin(phi))./(L_2.*(cos(alpha).*sin(phi)-cos(phi).*sin(alpha)))))./(L_3.*(cos(alpha).*sin(phi)-cos(phi).*sin(alpha)));
et63 = theta_dot.*cos(alpha).*cos(phi).*((L_1.*cos(alpha).*sin(theta))./(L_3.*(cos(alpha).*sin(phi)-cos(phi).*sin(alpha)))-(L_1.*sin(alpha).*cos(theta))./(L_3.*(cos(alpha).*sin(phi)-cos(phi).*sin(alpha))))-theta_dot.*cos(alpha).*cos(phi).*((L_1.*cos(phi).*sin(theta))./(L_2.*(cos(alpha).*sin(phi)-cos(phi).*sin(alpha)))-(L_1.*cos(theta).*sin(phi))./(L_2.*(cos(alpha).*sin(phi)-cos(phi).*sin(alpha))))+theta_dot.*sin(alpha).*sin(phi).*((L_1.*cos(alpha).*sin(theta))./(L_3.*(cos(alpha).*sin(phi)-cos(phi).*sin(alpha)))-(L_1.*sin(alpha).*cos(theta))./(L_3.*(cos(alpha).*sin(phi)-cos(phi).*sin(alpha))));
et64 = -theta_dot.*sin(alpha).*sin(phi).*((L_1.*cos(phi).*sin(theta))./(L_2.*(cos(alpha).*sin(phi)-cos(phi).*sin(alpha)))-(L_1.*cos(theta).*sin(phi))./(L_2.*(cos(alpha).*sin(phi)-cos(phi).*sin(alpha))));
et65 = theta_dot.*cos(alpha).*cos(phi).*((L_1.*cos(alpha).*sin(theta))./(L_3.*(cos(alpha).*sin(phi)-cos(phi).*sin(alpha)))-(L_1.*sin(alpha).*cos(theta))./(L_3.*(cos(alpha).*sin(phi)-cos(phi).*sin(alpha))))-theta_dot.*cos(alpha).*cos(phi).*((L_1.*cos(phi).*sin(theta))./(L_2.*(cos(alpha).*sin(phi)-cos(phi).*sin(alpha)))-(L_1.*cos(theta).*sin(phi))./(L_2.*(cos(alpha).*sin(phi)-cos(phi).*sin(alpha))))+theta_dot.*sin(alpha).*sin(phi).*((L_1.*cos(alpha).*sin(theta))./(L_3.*(cos(alpha).*sin(phi)-cos(phi).*sin(alpha)))-(L_1.*sin(alpha).*cos(theta))./(L_3.*(cos(alpha).*sin(phi)-cos(phi).*sin(alpha))));
et66 = -theta_dot.*sin(alpha).*sin(phi).*((L_1.*cos(phi).*sin(theta))./(L_2.*(cos(alpha).*sin(phi)-cos(phi).*sin(alpha)))-(L_1.*cos(theta).*sin(phi))./(L_2.*(cos(alpha).*sin(phi)-cos(phi).*sin(alpha))));
et67 = (L_1.*theta_dot.*cos(alpha).*cos(theta))./(L_3.*(cos(alpha).*sin(phi)-cos(phi).*sin(alpha)))+(L_1.*theta_dot.*sin(alpha).*sin(theta))./(L_3.*(cos(alpha).*sin(phi)-cos(phi).*sin(alpha)))-(L_1.*cos(alpha).*sin(theta).*1.0./(cos(alpha).*sin(phi)-cos(phi).*sin(alpha)).^2.*(et63+et64))./L_3+(L_1.*sin(alpha).*cos(theta).*1.0./(cos(alpha).*sin(phi)-cos(phi).*sin(alpha)).^2.*(et65+et66))./L_3-(L_1.*theta_dot.*cos(alpha).*cos(theta).*((L_1.*cos(phi).*sin(theta))./(L_2.*(cos(alpha).*sin(phi)-cos(phi).*sin(alpha)))-(L_1.*cos(theta).*sin(phi))./(L_2.*(cos(alpha).*sin(phi)-cos(phi).*sin(alpha)))))./(L_3.*(cos(alpha).*sin(phi)-cos(phi).*sin(alpha)));
et68 = -(L_1.*theta_dot.*sin(alpha).*sin(theta).*((L_1.*cos(phi).*sin(theta))./(L_2.*(cos(alpha).*sin(phi)-cos(phi).*sin(alpha)))-(L_1.*cos(theta).*sin(phi))./(L_2.*(cos(alpha).*sin(phi)-cos(phi).*sin(alpha)))))./(L_3.*(cos(alpha).*sin(phi)-cos(phi).*sin(alpha)));
et69 = -tau_1-(m_2.*(et16+et17))./2.0+(m_2.*(et30+et31+et32))./2.0+g.*m_2.*(L_1.*cos(theta)+(L_2.*cos(alpha).*((L_1.*cos(phi).*sin(theta))./(L_2.*(cos(alpha).*sin(phi)-cos(phi).*sin(alpha)))-(L_1.*cos(theta).*sin(phi))./(L_2.*(cos(alpha).*sin(phi)-cos(phi).*sin(alpha)))))./2.0)-I_G2.*theta_dot.^2.*((L_1.*cos(phi).*sin(theta))./(L_2.*(cos(alpha).*sin(phi)-cos(phi).*sin(alpha)))-(L_1.*cos(theta).*sin(phi))./(L_2.*(cos(alpha).*sin(phi)-cos(phi).*sin(alpha)))).*(et37+et38);
et70 = I_G2.*theta_dot.*((L_1.*cos(phi).*sin(theta))./(L_2.*(cos(alpha).*sin(phi)-cos(phi).*sin(alpha)))-(L_1.*cos(theta).*sin(phi))./(L_2.*(cos(alpha).*sin(phi)-cos(phi).*sin(alpha)))).*(et43+et44).*2.0+(L_1.*g.*m_1.*cos(theta))./2.0-I_G3.*theta_dot.^2.*((L_1.*cos(alpha).*sin(theta))./(L_3.*(cos(alpha).*sin(phi)-cos(phi).*sin(alpha)))-(L_1.*sin(alpha).*cos(theta))./(L_3.*(cos(alpha).*sin(phi)-cos(phi).*sin(alpha)))).*(et49+et50)+I_G3.*theta_dot.*((L_1.*cos(alpha).*sin(theta))./(L_3.*(cos(alpha).*sin(phi)-cos(phi).*sin(alpha)))-(L_1.*sin(alpha).*cos(theta))./(L_3.*(cos(alpha).*sin(phi)-cos(phi).*sin(alpha)))).*(et55+et56).*2.0;
et71 = (L_3.*g.*m_3.*cos(phi).*((L_1.*cos(alpha).*sin(theta))./(L_3.*(cos(alpha).*sin(phi)-cos(phi).*sin(alpha)))-(L_1.*sin(alpha).*cos(theta))./(L_3.*(cos(alpha).*sin(phi)-cos(phi).*sin(alpha)))))./2.0-(L_3.^2.*m_3.*theta_dot.^2.*((L_1.*cos(alpha).*sin(theta))./(L_3.*(cos(alpha).*sin(phi)-cos(phi).*sin(alpha)))-(L_1.*sin(alpha).*cos(theta))./(L_3.*(cos(alpha).*sin(phi)-cos(phi).*sin(alpha)))).*(et61+et62))./4.0;
et72 = (L_3.^2.*m_3.*theta_dot.*((L_1.*cos(alpha).*sin(theta))./(L_3.*(cos(alpha).*sin(phi)-cos(phi).*sin(alpha)))-(L_1.*sin(alpha).*cos(theta))./(L_3.*(cos(alpha).*sin(phi)-cos(phi).*sin(alpha)))).*(et67+et68))./2.0;
theta_DD = -(et69+et70+et71+et72)./(et1+et2+et3);

== matlab function bh_4bar_model_DYN/Hand_model_LAG_CONSTRAINTS_A_b/CHECK_CONSTRAINTS/MATLAB Function ==
  data: L_1 input; EQ_X output; L_2 input; L_3 input; L_4 input; THETA input; ALPHA input; PHI input; EQ_Y output
function [EQ_X, EQ_Y] = fcn(L_1, L_2, L_3, L_4,THETA, ALPHA, PHI)

   EQ_X = L_1*cos(THETA) + L_2*cos(ALPHA) - L_3*cos(PHI) - L_4;
   EQ_Y = L_1*sin(THETA) + L_2*sin(ALPHA) - L_3*sin(PHI);
end

== matlab function bh_4bar_model_DYN/Hand_model_LAG_CONSTRAINTS_A_b/CHECK_VELS_AGAINST_JACOBIANS/RATES_FROM_JACOBIANS ==
  data: theta_dot input; phi_dot output; theta input; phi input; alpha input; L1 input; L2 input; L3 input; alpha_dot output
function [phi_dot, alpha_dot] = LOC_calc_RATES_of_phi_alpha(theta_dot, theta, phi, alpha, L1, L2, L3)

    k = 1/(L3*L2*sin(phi)*cos(alpha) - L3*L2*cos(phi)*sin(alpha))

    A1 = [ -L2*cos(alpha),  -L2*sin(alpha);
           -L3*cos(phi),    -L3*sin(phi);   ];
       
    A2 = [-L1*sin(theta);
           L1*cos(theta) ];
       
   tmp_col   = k * A1 * A2 * theta_dot;
   
   phi_dot   = tmp_col(1);
   alpha_dot = tmp_col(2);
    
end

== matlab function bh_4bar_model_DYN/Hand_model_LAG_CONSTRAINTS_A_b/Hand_deriv_Lag/MATLAB Function ==
  data: A input; x output; b input
function x = fcn(A, b)

   x = zeros(5,1);

   x = A \ b;

end
